simulink model "MGS_linearizedInvertedPendulum_mdl"  (R2022b)
settings: Solver=ode4  StartTime=0.0  StopTime=.5  FixedStep=.001  RelTol=1e-3
undefined symbols (not defined in the file): G, SS_0
settings Model: Creator=mo780715  LastModifiedBy=mo780715

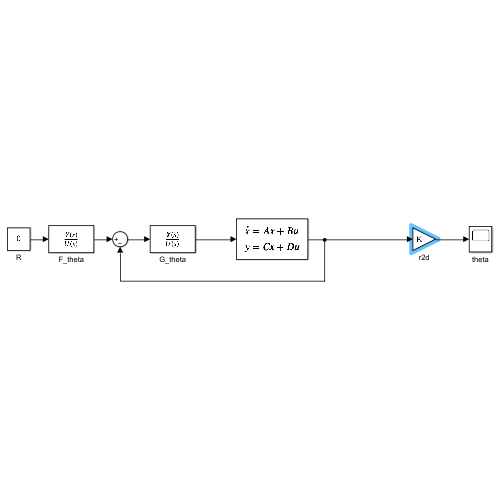
[thumbnail: Simulink's stored preview of the top-level diagram]
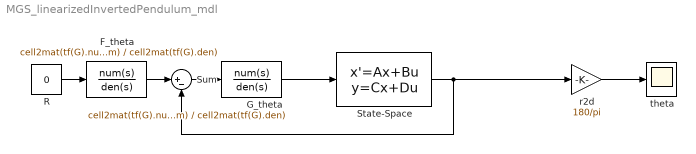
== system MGS_linearizedInvertedPendulum_mdl ==
  F_theta : TransferFcn  Numerator=cell2mat(tf(G).num)  Denominator=cell2mat(tf(G).den)
  G_theta : TransferFcn  Numerator=cell2mat(tf(G).num)  Denominator=cell2mat(tf(G).den)
  R : Constant  Value=0
  State-Space : StateSpace  A=SS_0.A  B=SS_0.B  C=SS_0.C  D=SS_0.D  InitialCondition=5/180*pi  ContinuousStateAttributes='theta'
  Sum : Sum  Inputs=|+-
  r2d : Gain  Gain=180/pi
  theta : Scope
  wires:
  r2d/1 -> theta/1
  State-Space/1 -> Sum/2, r2d/1
  G_theta/1 -> State-Space/1
  R/1 -> F_theta/1
  F_theta/1 -> Sum/1
  Sum/1 -> G_theta/1
